simulink model "SAC_RW"  (R2020b)
settings: Solver=ode4  StartTime=0.0  StopTime=T  FixedStep=s  RelTol=1e-3  EnableMultiTasking=on
values from neighbouring files (symbols this model uses):
  A = [zeros(3,3), eye(3); (-1*(wn)^2)*eye(3),-2*zeta*wn*eye(3)]    [ini_SAC.m]    (also in ini_SACRW.m = [zeros(3,3), eye(3); (-1*(wnn)^2)*eye(3),-2*zetaa*wnn*eye(3))
  a1_B = [1,0,0]'    [ini_SAC.m]    (also in ini_SACRW.m)
  a2_B = [0,1,0]'    [ini_SAC.m]    (also in ini_SACRW.m)
  a3_B = [0,0,1]'    [ini_SAC.m]    (also in ini_SACRW.m)
  alpha = 1    [ini_SAC.m]    (also in ini_SACRW.m)
  B = [zeros(3,3);(wn^2)*eye(3)]    [ini_SAC.m]    (also in ini_SACRW.m = [zeros(3,3);(wnn^2)*eye(3)])
  C = [eye(6)]    [ini_SAC.m]    (also in ini_SACRW.m)
  D = [zeros(6,3)]    [ini_SAC.m]    (also in ini_SACRW.m)
  gIE = 1e5*(eye(3))    [ini_SAC.m]    (also in ini_SACRW.m = 1e3*(eye(3)))
  gIU = 1e3*(eye(3))    [ini_SAC.m]    (also in ini_SACRW.m)
  gIX = 1e3*(eye(6))    [ini_SAC.m]    (also in ini_SACRW.m)
  gPE = 1e5*(eye(3))    [ini_SAC.m]    (also in ini_SACRW.m = 1e3*(eye(3)))
  gPU = 1e3*(eye(3))    [ini_SAC.m]    (also in ini_SACRW.m)
  gPX = 1e3*(eye(6))    [ini_SAC.m]    (also in ini_SACRW.m)
  Jsc = [114 0 0;0 86 0;0 0 87]    [ini_SAC.m]    (also in ini_SACRW.m = 1*[114 0 0;0 86 0;0 0 87])
  Jsc_inv = Jsc^-1    [ini_SAC.m]    (also in ini_SACRW.m)
  q_d = [0 0 0 1]'    [ini_SAC.m]    (also in ini_SACRW.m)
  qsc_I_ini = [a(1)*sin(phiR/2) a(2)*sin(phiR/2) a(3)*sin(phiR/2) cos(phiR/2)]    [ini_SACRW.m]
  r_I_ini = [-0.1 0.5 1.0]    [ini_SAC.m]
  r_I_ini_dot = [0 0 0]    [ini_SACRW.m]
  r_I_ini_pos = (qsc_I_ini(1:3)/qsc_I_ini(4))    [ini_SACRW.m]
  rw_t = 0.01    [ini_SAC.m]    (also in ini_SACRW.m)
undefined symbols (not defined in the file or in its folder): gammaE, gammaU, gammaX, K
libraries: simulink_extras x3
settings Model: Creator=hoomanrajaee  LastModifiedBy=Graham Stokes
settings DataIOCC: LimitDataPoints=on  SaveFormat=Array  SignalLoggingSaveFormat=ModelDataLogs  ReturnWorkspaceOutputs=off
settings OptimizationCC: LifeSpan=inf
settings DebuggingCC: UnderspecifiedInitializationDetection=Classic  MergeDetectMultiDrivingBlocksExec=none  SolverPrmCheckMsg=warning  MultiTaskDSMMsg=warning  MultiTaskCondExecSysMsg=none  AllowSymbolicDim=off  StateNameClashWarn=warning  SFUnexpectedBacktrackingDiag=warning  SFNoUnconditionalDefaultTransitionDiag=warning  UnderSpecifiedDimensionMsg=warning  ArithmeticOperatorsInVariantConditions=warning
settings HardwareCC: ProdBitPerPointer=32  ProdBitPerSizeT=32  ProdBitPerPtrDiffT=32  ProdLargestAtomicFloat=None  ProdIntDivRoundTo=Undefined  ProdEndianess=Unspecified  ProdWordSize=32  ProdHWDeviceType=32-bit Generic
settings ModelReferenceCC: PropagateSignalLabelsOutOfModel=off
settings SFSimCC: SimUseLocalCustomCode=off  CustomCodeUndefinedFunction=UseInterfaceOnly
settings RTWCC: RTWUseLocalCustomCode=off
settings CodeAppCC: StateflowObjectComments=on
settings GRTTargetCC: TargetLangStandard=C89/C90 (ANSI)
settings ConfigComp: CovMetricSettings=dw  CovSaveCumulativeToWorkspaceVar=on  CovSaveSingleToWorkspaceVar=on  CovExternalEMLEnable=off

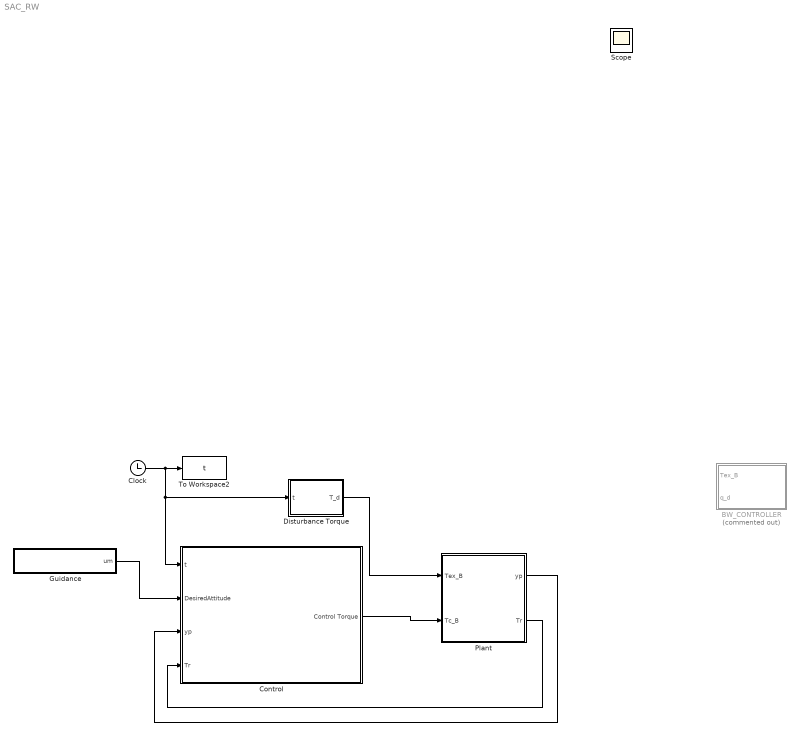
== system SAC_RW ==
  BW_CONTROLLER : Subsystem  Commented=on
  Clock : Clock
  Control : Subsystem
  Disturbance Torque : MATLAB Function  TreatAsAtomicUnit=on
  "Guidance " : Subsystem
  Plant : Subsystem
  To Workspace2 : ToWorkspace  VariableName=t  SampleTime=-1
  Scope : Scope
  wires:
  Clock/1 -> Disturbance Torque/1(t), Control/1(t), To Workspace2/1
  "Guidance "/1(um) -> Control/2(DesiredAttitude)
  Control/1(Control Torque) -> Plant/2(Tc_B)
  Plant/1("yp ") -> Control/3(yp)
  Plant/2("Tr ") -> Control/4(Tr)
  Disturbance Torque/1(T_d) -> Plant/1(Tex_B)

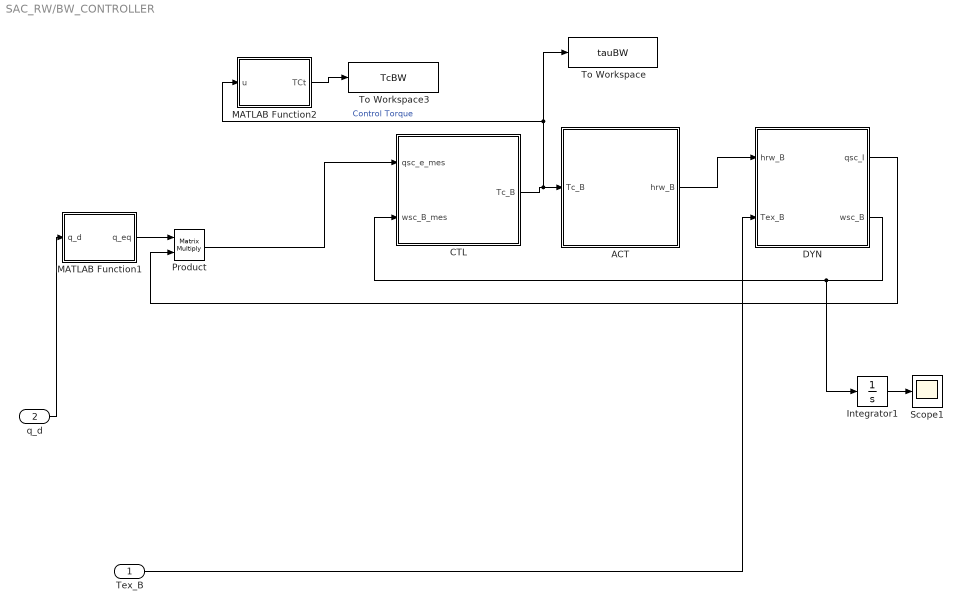
== system SAC_RW/BW_CONTROLLER ==
  Tex_B : Inport
  q_d : Inport  Port=2
  ACT : Subsystem
  CTL : Subsystem
  DYN : Subsystem
  Integrator1 : Integrator  InitialCondition=r_I_ini
  MATLAB Function1 : MATLAB Function  TreatAsAtomicUnit=on
  MATLAB Function2 : MATLAB Function  TreatAsAtomicUnit=on
  Product : Product  Multiplication=Matrix(*)
  Scope1 : Scope
  To Workspace : ToWorkspace  VariableName=tauBW  SaveFormat=Timeseries  SampleTime=-1
  To Workspace3 : ToWorkspace  VariableName=TcBW  SaveFormat=Timeseries  SampleTime=-1
  wires:
  ACT/1(hrw_B) -> DYN/1(hrw_B)
  MATLAB Function1/1(q_eq) -> Product/1
  DYN/1(qsc_I) -> Product/2
  Product/1 -> CTL/1(qsc_e_mes)
  q_d/1 -> MATLAB Function1/1(q_d)
  Tex_B/1 -> DYN/2(Tex_B)
  CTL/1(Tc_B) -> To Workspace/1, MATLAB Function2/1(u), ACT/1(Tc_B)  "Control Torque"
  MATLAB Function2/1(TCt) -> To Workspace3/1
  Integrator1/1 -> Scope1/1
  DYN/2(wsc_B) -> Integrator1/1, CTL/2(wsc_B_mes)

== system SAC_RW/Control ==
  t : Inport
  DesiredAttitude : Inport  Port=2
  yp : Inport  Port=3
  Tr : Inport  Port=4
  ADAPTIVE CONTROLLER : Subsystem
      settings: AttributesFormatString=Adaptive Controller
  MODEL PLANT : Subsystem
  Sum : Sum  Inputs=|+-
  To Workspace : ToWorkspace  VariableName=tau  SaveFormat=Timeseries  SampleTime=-1
  Control Torque : Outport
  wires:
  DesiredAttitude/1 -> ADAPTIVE CONTROLLER/4(um1), MODEL PLANT/1(DesiredAttitude)
  MODEL PLANT/2(ym) -> Sum/1
  Tr/1 -> ADAPTIVE CONTROLLER/2(Tr)
  ADAPTIVE CONTROLLER/1(tau) -> To Workspace/1, Control Torque/1  "Control Torque"
  yp/1 -> Sum/2
  Sum/1 -> ADAPTIVE CONTROLLER/1(ey1)  "ey"
  MODEL PLANT/1(xm) -> ADAPTIVE CONTROLLER/3(xm1)
  t/1 -> MODEL PLANT/2(In2)

== system SAC_RW/Guidance  ==
  MRP : MATLAB Function  TreatAsAtomicUnit=on
  To Workspace : ToWorkspace  VariableName=um  SaveFormat=Timeseries  SampleTime=-1
  q_d1 : Constant  Value=q_d
  um : Outport
  wires:
  MRP/1(r) -> To Workspace/1, um/1  "um"
  q_d1/1 -> MRP/1(qsc_I_sign)

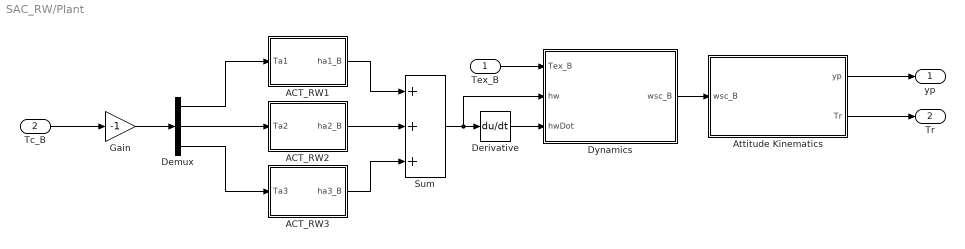
== system SAC_RW/Plant ==
  Tex_B : Inport
  Tc_B : Inport  Port=2
  ACT_RW1 : Subsystem
  ACT_RW2 : Subsystem
  ACT_RW3 : Subsystem
  Attitude Kinematics : Subsystem
  Demux : Demux  Outputs=3
  Derivative : Derivative
  Dynamics : Subsystem
  Gain : Gain  Gain=-1
  Sum : Sum  Inputs=+++
  "yp " : Outport
  "Tr " : Outport  Port=2
  wires:
  Attitude Kinematics/2(Tr) -> "Tr "/1
  Attitude Kinematics/1(yp) -> "yp "/1
  Demux/3 -> ACT_RW3/1(Ta3)
  ACT_RW2/1(ha2_B) -> Sum/2
  Demux/1 -> ACT_RW1/1(Ta1)
  ACT_RW1/1(ha1_B) -> Sum/1
  ACT_RW3/1(ha3_B) -> Sum/3
  Sum/1 -> Derivative/1, Dynamics/2(hw)
  Demux/2 -> ACT_RW2/1(Ta2)
  Derivative/1 -> Dynamics/3(hwDot)
  Tex_B/1 -> Dynamics/1(Tex_B)
  Tc_B/1 -> Gain/1
  Dynamics/1(wsc_B) -> Attitude Kinematics/1(wsc_B)
  Gain/1 -> Demux/1

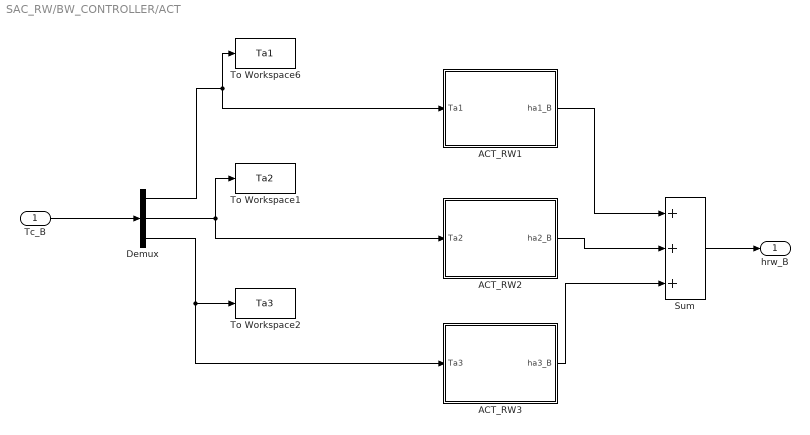
== system SAC_RW/BW_CONTROLLER/ACT ==
  Tc_B : Inport
  ACT_RW1 : Subsystem
  ACT_RW2 : Subsystem
  ACT_RW3 : Subsystem
  Demux : Demux  Outputs=3
  Sum : Sum  Inputs=+++
  To Workspace1 : ToWorkspace  VariableName=Ta2  SampleTime=-1
  To Workspace2 : ToWorkspace  VariableName=Ta3  SampleTime=-1
  To Workspace6 : ToWorkspace  VariableName=Ta1  SampleTime=-1
  hrw_B : Outport
  wires:
  ACT_RW1/1(ha1_B) -> Sum/1
  Sum/1 -> hrw_B/1
  Demux/1 -> ACT_RW1/1(Ta1), To Workspace6/1
  Demux/2 -> To Workspace1/1, ACT_RW2/1(Ta2)
  Demux/3 -> To Workspace2/1, ACT_RW3/1(Ta3)
  ACT_RW2/1(ha2_B) -> Sum/2
  ACT_RW3/1(ha3_B) -> Sum/3
  Tc_B/1 -> Demux/1

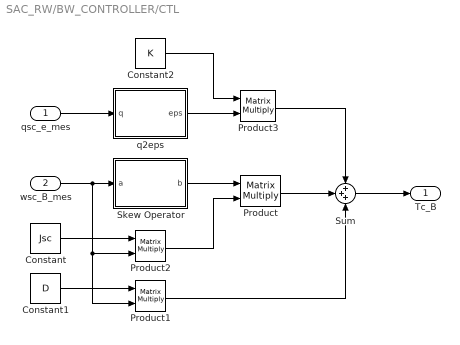
== system SAC_RW/BW_CONTROLLER/CTL ==
  qsc_e_mes : Inport
  wsc_B_mes : Inport  Port=2
  Constant : Constant  Value=Jsc
  Constant1 : Constant  Value=D
  Constant2 : Constant  Value=K
  Product{,1..3} (4 alike) : Product  Multiplication=Matrix(*)
  Skew Operator : MATLAB Function  TreatAsAtomicUnit=on
  Sum : Sum  Inputs=+++
  q2eps : MATLAB Function  TreatAsAtomicUnit=on
  Tc_B : Outport
  wires:
  wsc_B_mes/1 -> Skew Operator/1(a), Product2/2, Product1/2
  Skew Operator/1(b) -> Product/1
  Product2/1 -> Product/2
  Product3/1 -> Sum/1
  qsc_e_mes/1 -> q2eps/1(q)
  q2eps/1(eps) -> Product3/2
  Sum/1 -> Tc_B/1
  Product1/1 -> Sum/3
  Constant/1 -> Product2/1
  Constant1/1 -> Product1/1
  Constant2/1 -> Product3/1
  Product/1 -> Sum/2

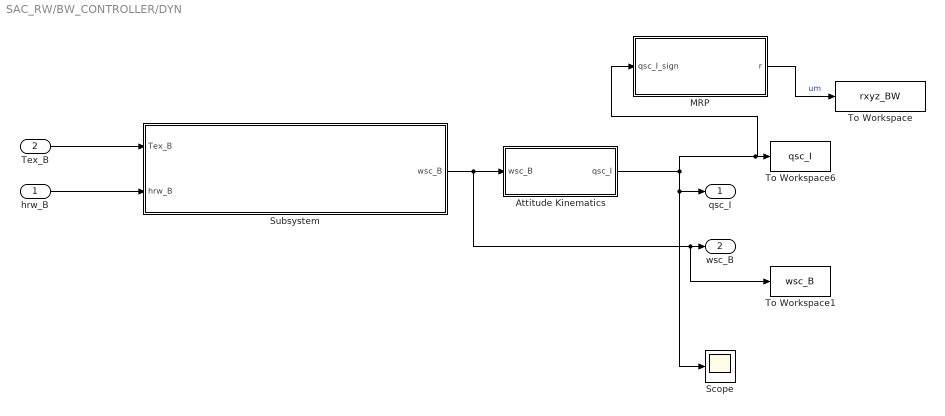
== system SAC_RW/BW_CONTROLLER/DYN ==
  hrw_B : Inport
  Tex_B : Inport  Port=2
  Attitude Kinematics : Subsystem
  MRP : MATLAB Function  TreatAsAtomicUnit=on
  Scope : Scope
  Subsystem : Subsystem
  To Workspace : ToWorkspace  VariableName=rxyz_BW  SaveFormat=Timeseries  SampleTime=-1
  To Workspace1 : ToWorkspace  VariableName=wsc_B  SampleTime=-1
  To Workspace6 : ToWorkspace  VariableName=qsc_I  SampleTime=-1
  qsc_I : Outport
  wsc_B : Outport  Port=2
  wires:
  Attitude Kinematics/1(qsc_I) -> Scope/1, qsc_I/1, MRP/1(qsc_I_sign), To Workspace6/1
  Subsystem/1(wsc_B) -> To Workspace1/1, wsc_B/1, Attitude Kinematics/1(wsc_B)
  Tex_B/1 -> Subsystem/1(Tex_B)
  hrw_B/1 -> Subsystem/2(hrw_B)
  MRP/1(r) -> To Workspace/1  "um"

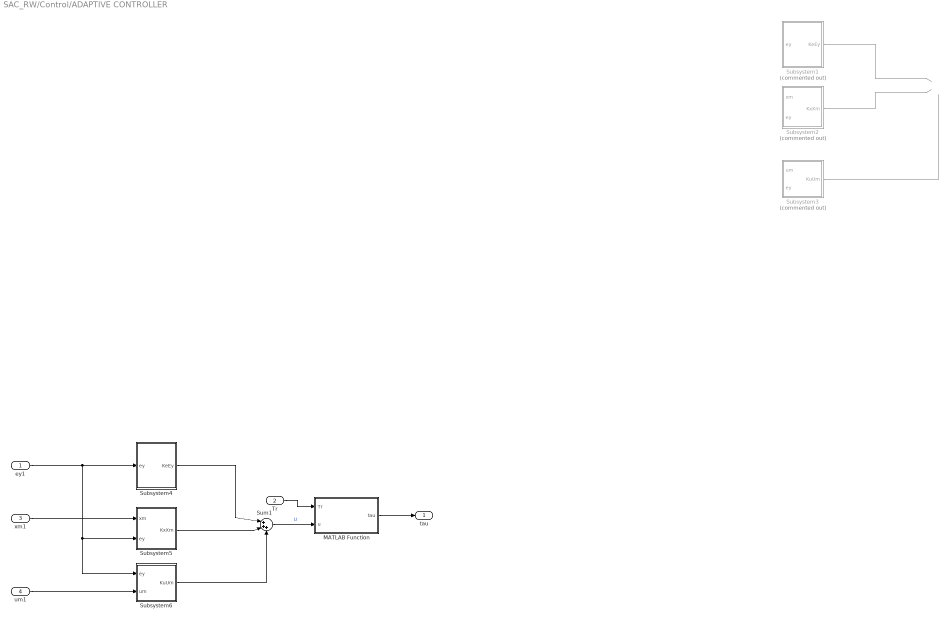
== system SAC_RW/Control/ADAPTIVE CONTROLLER ==
  ey1 : Inport
  Tr : Inport  Port=2
  xm1 : Inport  Port=3
  um1 : Inport  Port=4
  MATLAB Function : MATLAB Function  TreatAsAtomicUnit=on
  Subsystem1 : Subsystem  Commented=on
  Subsystem2 : Subsystem  Commented=on
  Subsystem3 : Subsystem  Commented=on
  Subsystem4 : Subsystem
  Subsystem5 : Subsystem
  Subsystem6 : Subsystem
  Sum1 : Sum  Inputs=|+++
  tau : Outport
  wires:
  Tr/1 -> MATLAB Function/1(Tr)
  Sum1/1 -> MATLAB Function/2(u)  "U"
  MATLAB Function/1(tau) -> tau/1
  Subsystem5/1(KxXm) -> Sum1/2
  Subsystem4/1(KeEy) -> Sum1/1
  Subsystem6/1(KuUm) -> Sum1/3
  um1/1 -> Subsystem6/2(um)
  xm1/1 -> Subsystem5/1(xm)
  ey1/1 -> Subsystem4/1(ey), Subsystem6/1(ey), Subsystem5/2(ey)
  Subsystem2/1(KxXm) -> ?
  Subsystem3/1(KuUm) -> ?
  Subsystem1/1(KeEy) -> ?

== system SAC_RW/Control/MODEL PLANT ==
  DesiredAttitude : Inport
  In2 : Inport  Port=2
  Constant : Constant  Value=alpha
  MATLAB Function : MATLAB Function  TreatAsAtomicUnit=on
  Scope : Scope
  State Space Model : Subsystem
  State-Space : StateSpace  Commented=on  A=A  B=B  C=C  D=D  InitialCondition=[r_I_ini(1);r_I_ini(2);r_I_ini(3);0;0;0]
  xm : Outport
  ym : Outport  Port=2
  wires:
  MATLAB Function/1(ym) -> ym/1
  Constant/1 -> MATLAB Function/2(alpha)
  State Space Model/1(Xm) -> xm/1, Scope/1, MATLAB Function/1(Xm)
  DesiredAttitude/1 -> State Space Model/1(DesiredAttitude)  "U"
  In2/1 -> State Space Model/2(In2)

== system SAC_RW/Plant/ACT_RW1 ==
  Ta1 : Inport
  Constant1 : Constant  Value=a1_B
  Integrator : Integrator
  Product1 : Product
  Transfer Fcn (with initial states) : simulink_extras/Additional Linear/Transfer Fcn (with initial states)  N=[1]  D=[rw_t 1]  X0=.5
  ha1_B : Outport
  wires:
  Product1/1 -> ha1_B/1
  Integrator/1 -> Product1/1
  Constant1/1 -> Product1/2
  Ta1/1 -> Transfer Fcn (with initial states)/1
  Transfer Fcn (with initial states)/1 -> Integrator/1

== system SAC_RW/Plant/ACT_RW2 ==
  Ta2 : Inport
  Constant1 : Constant  Value=a2_B
  Integrator : Integrator
  Product1 : Product
  Transfer Fcn (with initial states) : simulink_extras/Additional Linear/Transfer Fcn (with initial states)  N=[1]  D="[rw_t  1]"  X0=.5
  ha2_B : Outport
  wires:
  Constant1/1 -> Product1/2
  Product1/1 -> ha2_B/1
  Integrator/1 -> Product1/1
  Ta2/1 -> Transfer Fcn (with initial states)/1  "Tcmd"
  Transfer Fcn (with initial states)/1 -> Integrator/1

== system SAC_RW/Plant/ACT_RW3 ==
  Ta3 : Inport
  Constant1 : Constant  Value=a3_B
  Integrator : Integrator
  Product1 : Product
  Transfer Fcn (with initial states) : simulink_extras/Additional Linear/Transfer Fcn (with initial states)  N=[1]  D="[rw_t  1]"  X0=.5
  ha3_B : Outport
  wires:
  Constant1/1 -> Product1/2
  Product1/1 -> ha3_B/1
  Integrator/1 -> Product1/1
  Ta3/1 -> Transfer Fcn (with initial states)/1  "Tcmd"
  Transfer Fcn (with initial states)/1 -> Integrator/1

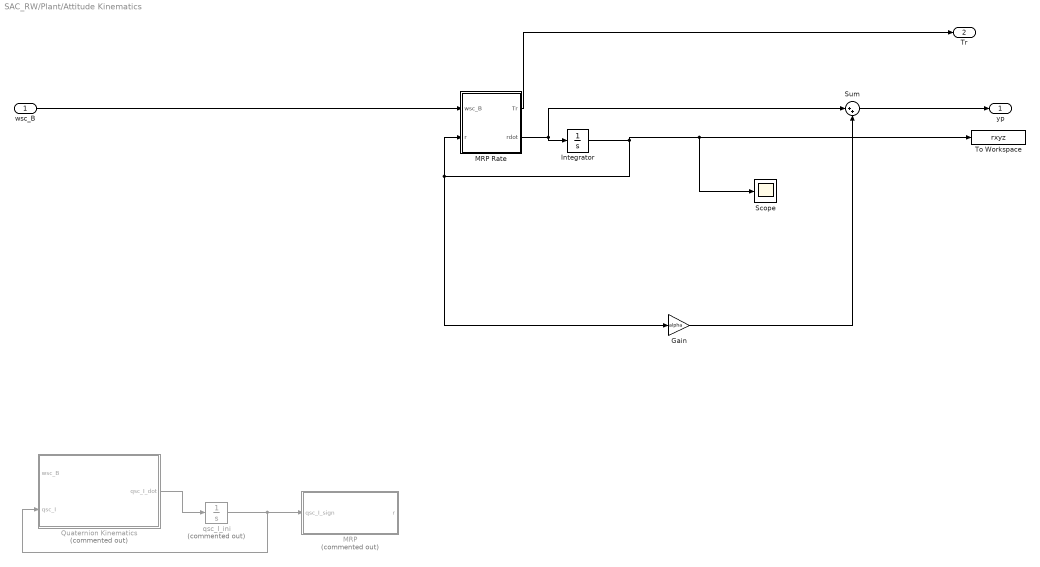
== system SAC_RW/Plant/Attitude Kinematics ==
  wsc_B : Inport
  Gain : Gain  Gain=alpha
  Integrator : Integrator  InitialCondition=r_I_ini_pos
  MRP : MATLAB Function  Commented=on  TreatAsAtomicUnit=on
  MRP Rate : MATLAB Function  TreatAsAtomicUnit=on
  Quaternion Kinematics : MATLAB Function  Commented=on  TreatAsAtomicUnit=on
  Scope : Scope
  Sum : Sum  Inputs=|++
  To Workspace : ToWorkspace  VariableName=rxyz  SaveFormat=Timeseries  SampleTime=-1
  qsc_I_ini : Integrator  Commented=on  InitialCondition=qsc_I_ini
  yp : Outport
  Tr : Outport  Port=2
  wires:
  MRP Rate/2(rdot) -> Sum/1, Integrator/1
  Sum/1 -> yp/1
  Gain/1 -> Sum/2
  MRP Rate/1(Tr) -> Tr/1
  wsc_B/1 -> MRP Rate/1(wsc_B)
  Quaternion Kinematics/1(qsc_I_dot) -> qsc_I_ini/1
  qsc_I_ini/1 -> MRP/1(qsc_I_sign), Quaternion Kinematics/2(qsc_I)
  Integrator/1 -> Gain/1, MRP Rate/2(r), Scope/1, To Workspace/1

== system SAC_RW/Plant/Dynamics ==
  Tex_B : Inport
  hw : Inport  Port=2
  hwDot : Inport  Port=3
  Constant1 : Constant  Value=Jsc
  Integrator : Integrator  InitialCondition=[0 0 0]';
  MATLAB Function : MATLAB Function  TreatAsAtomicUnit=on
  To Workspace : ToWorkspace  VariableName=w_sc  SaveFormat=Timeseries  SampleTime=-1
  wsc_B : Outport
  wires:
  Integrator/1 -> MATLAB Function/2(wsc_B), To Workspace/1, wsc_B/1
  Constant1/1 -> MATLAB Function/3(Jsc)
  MATLAB Function/1(angularAcceleration) -> Integrator/1
  Tex_B/1 -> MATLAB Function/1(Tex_B)
  hw/1 -> MATLAB Function/4(hw)
  hwDot/1 -> MATLAB Function/5(hwDot)

== system SAC_RW/BW_CONTROLLER/ACT/ACT_RW1 ==
  Ta1 : Inport
  Constant1 : Constant  Value=a1_B
  Integrator : Integrator
  Product1 : Product
  ha1_B : Outport
  wires:
  Ta1/1 -> Integrator/1
  Product1/1 -> ha1_B/1
  Integrator/1 -> Product1/1
  Constant1/1 -> Product1/2

== system SAC_RW/BW_CONTROLLER/ACT/ACT_RW2 ==
  Ta2 : Inport
  Constant1 : Constant  Value=a2_B
  Integrator : Integrator
  Product1 : Product
  ha2_B : Outport
  wires:
  Constant1/1 -> Product1/2
  Product1/1 -> ha2_B/1
  Integrator/1 -> Product1/1
  Ta2/1 -> Integrator/1

== system SAC_RW/BW_CONTROLLER/ACT/ACT_RW3 ==
  Ta3 : Inport
  Constant1 : Constant  Value=a3_B
  Integrator : Integrator
  Product1 : Product
  ha3_B : Outport
  wires:
  Constant1/1 -> Product1/2
  Product1/1 -> ha3_B/1
  Integrator/1 -> Product1/1
  Ta3/1 -> Integrator/1

== system SAC_RW/BW_CONTROLLER/DYN/Attitude Kinematics ==
  wsc_B : Inport
  Quaternion Kinematics : MATLAB Function  TreatAsAtomicUnit=on
  Quaternion Normalization : MATLAB Function  TreatAsAtomicUnit=on
  Quaternion Sign Check : MATLAB Function  TreatAsAtomicUnit=on
  qsc_I_ini : Integrator  InitialCondition=qsc_I_ini
  qsc_I : Outport
  wires:
  Quaternion Kinematics/1(qsc_I_dot) -> qsc_I_ini/1
  wsc_B/1 -> Quaternion Kinematics/1(wsc_B)
  Quaternion Sign Check/1(qsc_I_sign) -> Quaternion Kinematics/2(qsc_I), qsc_I/1
  Quaternion Normalization/1(qsc_I_norm) -> Quaternion Sign Check/1(qsc_I)
  qsc_I_ini/1 -> Quaternion Normalization/1(qsc_I)

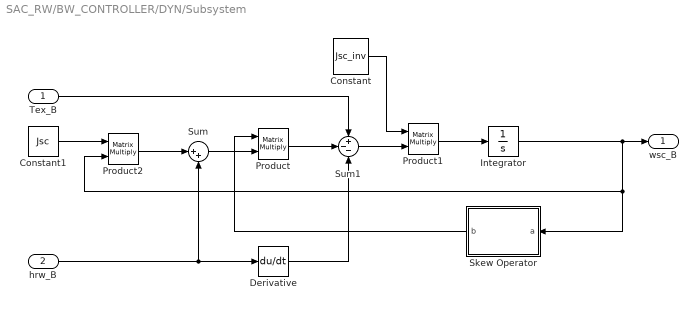
== system SAC_RW/BW_CONTROLLER/DYN/Subsystem ==
  Tex_B : Inport
  hrw_B : Inport  Port=2
  Constant : Constant  Value=Jsc_inv
  Constant1 : Constant  Value=Jsc
  Derivative : Derivative
  Integrator : Integrator
  Product : Product  Multiplication=Matrix(*)
  Product1 : Product  Multiplication=Matrix(*)
  Product2 : Product  Multiplication=Matrix(*)
  Skew Operator : MATLAB Function  TreatAsAtomicUnit=on
  Sum : Sum  Inputs=|++
  Sum1 : Sum  Inputs=+--
  wsc_B : Outport
  wires:
  hrw_B/1 -> Derivative/1, Sum/2
  Integrator/1 -> wsc_B/1, Skew Operator/1(a), Product2/2
  Product2/1 -> Sum/1
  Product/1 -> Sum1/2
  Derivative/1 -> Sum1/3
  Tex_B/1 -> Sum1/1
  Product1/1 -> Integrator/1
  Sum1/1 -> Product1/2
  Constant/1 -> Product1/1
  Skew Operator/1(b) -> Product/1
  Sum/1 -> Product/2
  Constant1/1 -> Product2/1

== system SAC_RW/Control/ADAPTIVE CONTROLLER/Subsystem1 ==
  ey : Inport
  Add : Sum
  Constant1 : Constant  Value=gammaE
  Integrator : Integrator
  KIE : MATLAB Function  TreatAsAtomicUnit=on
  KPE : MATLAB Function  TreatAsAtomicUnit=on
  MATLAB Function : MATLAB Function  Commented=on  TreatAsAtomicUnit=on
  Product : Product  Multiplication=Matrix(*)
  KeEy : Outport
  wires:
  ey/1 -> Product/2, KPE/1(ey), KIE/1(ey)
  KPE/1(Kpe) -> Add/1
  KIE/1(KIe) -> Integrator/1
  Constant1/1 -> KPE/2(gammaE), KIE/2(gammaE)
  Product/1 -> KeEy/1  "KeEy"
  Integrator/1 -> Add/2
  Add/1 -> Product/1

== system SAC_RW/Control/ADAPTIVE CONTROLLER/Subsystem2 ==
  xm : Inport
  ey : Inport  Port=2
  Add : Sum
  Constant1 : Constant  Value=gammaX
  Integrator : Integrator
  KIX : MATLAB Function  TreatAsAtomicUnit=on
  KPE : MATLAB Function  TreatAsAtomicUnit=on
  MATLAB Function : MATLAB Function  Commented=on  TreatAsAtomicUnit=on
  Product : Product  Multiplication=Matrix(*)
  KxXm : Outport
  wires:
  ey/1 -> KPE/1(ey), KIX/1(ey)
  xm/1 -> Product/2, KIX/2(xm), KPE/2(xm)
  Add/1 -> Product/1
  Integrator/1 -> Add/2
  KPE/1(Kpx) -> Add/1
  Constant1/1 -> KPE/3(gammaX), KIX/3(gammaX)
  Product/1 -> KxXm/1  "KXxm"
  KIX/1(KIx) -> Integrator/1

== system SAC_RW/Control/ADAPTIVE CONTROLLER/Subsystem3 ==
  um : Inport
  ey : Inport  Port=2
  Add : Sum
  Constant1 : Constant  Value=gammaU
  Integrator : Integrator
  KIu : MATLAB Function  TreatAsAtomicUnit=on
  KPE : MATLAB Function  TreatAsAtomicUnit=on
  MATLAB Function : MATLAB Function  Commented=on  TreatAsAtomicUnit=on
  Product : Product  Multiplication=Matrix(*)
  KuUm : Outport
  wires:
  Product/1 -> KuUm/1  "KuUm"
  KIu/1(KIu) -> Integrator/1
  ey/1 -> KPE/1(ey), KIu/1(ey)
  KPE/1(KPu) -> Add/1
  Integrator/1 -> Add/2
  Constant1/1 -> KIu/3(gammaU), KPE/3(gammaU)
  um/1 -> Product/2, KPE/2(um), KIu/2(um)
  Add/1 -> Product/1

== system SAC_RW/Control/ADAPTIVE CONTROLLER/Subsystem4 ==
  ey : Inport
  Add : Sum
  Constant1 : Constant  Value=gPE
  Constant2 : Constant  Value=gIE
  Integrator : Integrator
  KIE : MATLAB Function  TreatAsAtomicUnit=on
  KPE : MATLAB Function  TreatAsAtomicUnit=on
  Product : Product  Multiplication=Matrix(*)
  KeEy : Outport
  wires:
  ey/1 -> KPE/1(ey), KIE/1(ey), Product/2
  KPE/1(Kpe) -> Add/1
  KIE/1(KIe) -> Integrator/1
  Constant1/1 -> KPE/2(gPE)
  Product/1 -> KeEy/1  "KeEy"
  Integrator/1 -> Add/2
  Add/1 -> Product/1
  Constant2/1 -> KIE/2(gIE)

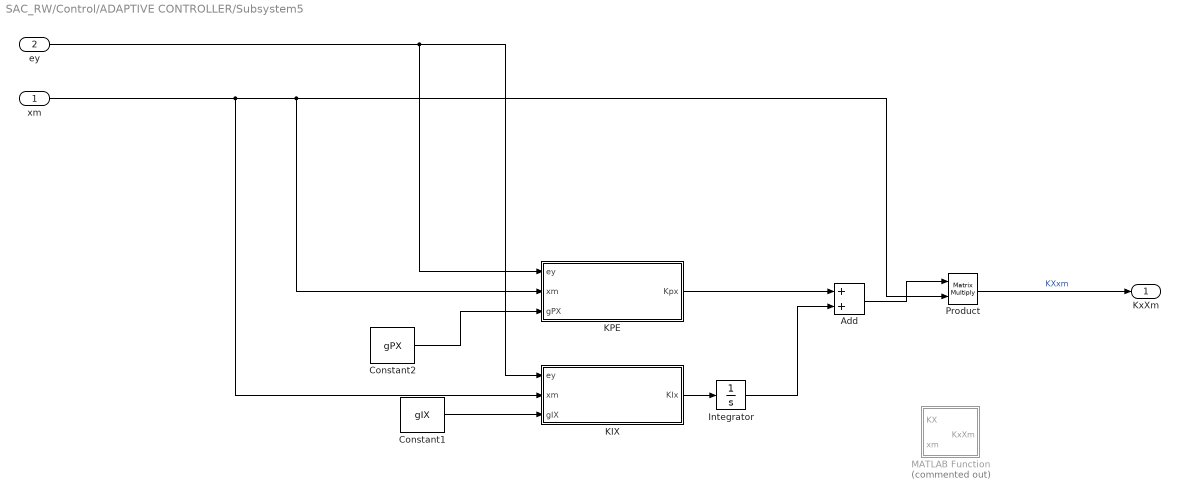
== system SAC_RW/Control/ADAPTIVE CONTROLLER/Subsystem5 ==
  xm : Inport
  ey : Inport  Port=2
  Add : Sum
  Constant1 : Constant  Value=gIX
  Constant2 : Constant  Value=gPX
  Integrator : Integrator
  KIX : MATLAB Function  TreatAsAtomicUnit=on
  KPE : MATLAB Function  TreatAsAtomicUnit=on
  MATLAB Function : MATLAB Function  Commented=on  TreatAsAtomicUnit=on
  Product : Product  Multiplication=Matrix(*)
  KxXm : Outport
  wires:
  ey/1 -> KPE/1(ey), KIX/1(ey)
  xm/1 -> KPE/2(xm), Product/2, KIX/2(xm)
  Add/1 -> Product/1
  Integrator/1 -> Add/2
  KPE/1(Kpx) -> Add/1
  Constant1/1 -> KIX/3(gIX)
  Product/1 -> KxXm/1  "KXxm"
  KIX/1(KIx) -> Integrator/1
  Constant2/1 -> KPE/3(gPX)

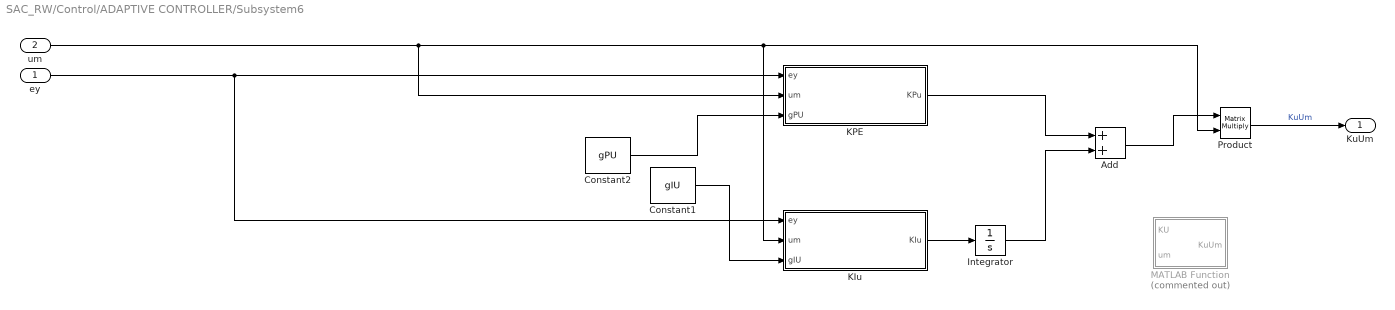
== system SAC_RW/Control/ADAPTIVE CONTROLLER/Subsystem6 ==
  ey : Inport
  um : Inport  Port=2
  Add : Sum
  Constant1 : Constant  Value=gIU
  Constant2 : Constant  Value=gPU
  Integrator : Integrator
  KIu : MATLAB Function  TreatAsAtomicUnit=on
  KPE : MATLAB Function  TreatAsAtomicUnit=on
  MATLAB Function : MATLAB Function  Commented=on  TreatAsAtomicUnit=on
  Product : Product  Multiplication=Matrix(*)
  KuUm : Outport
  wires:
  Product/1 -> KuUm/1  "KuUm"
  KIu/1(KIu) -> Integrator/1
  ey/1 -> KPE/1(ey), KIu/1(ey)
  KPE/1(KPu) -> Add/1
  Integrator/1 -> Add/2
  Constant1/1 -> KIu/3(gIU)
  um/1 -> KIu/2(um), Product/2, KPE/2(um)
  Add/1 -> Product/1
  Constant2/1 -> KPE/3(gPU)

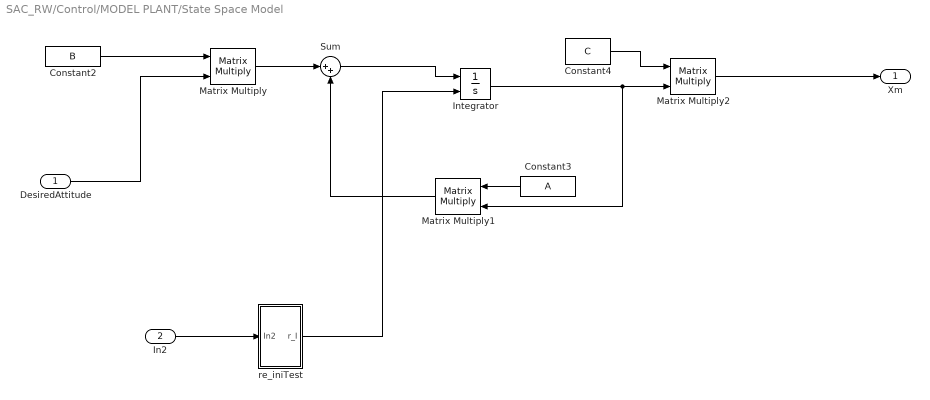
== system SAC_RW/Control/MODEL PLANT/State Space Model ==
  DesiredAttitude : Inport
  In2 : Inport  Port=2
  Constant2 : Constant  Value=B
  Constant3 : Constant  Value=A
  Constant4 : Constant  Value=C
  Integrator : Integrator  InitialConditionSource=external
  Matrix Multiply : Product  Multiplication=Matrix(*)
  Matrix Multiply1 : Product  Multiplication=Matrix(*)
  Matrix Multiply2 : Product  Multiplication=Matrix(*)
  Sum : Sum  Inputs=|++
  re_iniTest : Subsystem
  Xm : Outport
  wires:
  Matrix Multiply/1 -> Sum/1
  Integrator/1 -> Matrix Multiply2/2, Matrix Multiply1/2
  Sum/1 -> Integrator/1
  DesiredAttitude/1 -> Matrix Multiply/2
  Constant4/1 -> Matrix Multiply2/1
  Constant2/1 -> Matrix Multiply/1
  Matrix Multiply1/1 -> Sum/2
  Constant3/1 -> Matrix Multiply1/1
  Matrix Multiply2/1 -> Xm/1
  In2/1 -> re_iniTest/1(In2)
  re_iniTest/1(r_I) -> Integrator/2

== system SAC_RW/Control/MODEL PLANT/State Space Model/re_iniTest ==
  In2 : Inport
  Constant1 : Constant  Value=r_I_ini_pos
  Constant5 : Constant  Value=r_I_ini_dot
  MATLAB Function : MATLAB Function  TreatAsAtomicUnit=on
  r_I : Outport
  wires:
  In2/1 -> MATLAB Function/1(t)
  Constant1/1 -> MATLAB Function/2(r_I_ini_pos)
  MATLAB Function/1(r_I) -> r_I/1
  Constant5/1 -> MATLAB Function/3(r_I_ini_dot)

== matlab function SAC_RW/Control/MODEL PLANT/MATLAB Function ==
  data: Xm input; ym output; alpha input
function ym = parseY(Xm, alpha)
    
    %creates a 3X1 matrix of state output
    %Includes position and damping value--> similar to plant output
    ym = alpha*eye(3)*Xm(1:3) + Xm(4:6);
    
end

== matlab function SAC_RW/Control/ADAPTIVE CONTROLLER/Subsystem3/MATLAB Function ==
  data: KU input; um input; KuUm output
function  KuUm = fcn(KU, um)

KuUm = KU*um

end

== matlab function SAC_RW/Control/ADAPTIVE CONTROLLER/Subsystem2/MATLAB Function ==
  data: KX input; xm input; KxXm output
function  KxXm = KX(KX, xm)

KxXm = KX*xm

end

== matlab function SAC_RW/Plant/Attitude Kinematics/MRP ==
  data: qsc_I_sign input; r output
function r  = QuatToMRP(qsc_I_sign)
    q = qsc_I_sign; 
    r = zeros(3,1); 
    eps = zeros(3,1); 
    
    eps(1) = q(1);
    eps(2) = q(2); 
    eps(3) = q(3); 
    
    r = eps/(1+q(4)); 
end

== matlab function SAC_RW/Plant/Attitude Kinematics/MRP Rate ==
  data: Tr output; wsc_B input; r input; rdot output
function [Tr,rdot]= fcn(wsc_B,r)
        
    Tr = zeros(3,3); 
    Tr = 0.25*((1-transpose(r)*r)*eye(3)+2*skew(r)+2*r*transpose(r));
   
    TrInv = zeros(3,3); 
    TrInv = 4*(((1+transpose(r)*r)^-2)*(1-transpose(r)*r)*eye(3)-2*skew(r)+2*r*transpose(r));
    
    %set size of T(r) matrix 
    rdot = Tr*wsc_B; 
    
end

== matlab function SAC_RW/Plant/Attitude Kinematics/Quaternion Kinematics ==
  data: wsc_B input; qsc_I_dot output; qsc_I input
function qsc_I_dot  = qdot(wsc_B,qsc_I)

% ---------------------------------------------------------------
% qdot
% ---------------------------------------------------------------
% Description:
% Calculate the quaternion differential kinematics
% ---------------------------------------------------------------
% Inputs:
% qsc_I => quaternion (4 x 1 matrix)
% wsc_B => angular rates (3 x 1 matrix)
% ---------------------------------------------------------------
% Outputs:
% qsc_I_dot => quaternion derivatives (4 x 1 matrix) 
% ---------------------------------------------------------------
% Parameters:
% None
% ---------------------------------------------------------------
% Copyright:
% Steve Ulrich, 2020
% ---------------------------------------------------------------

%prealocating
qsc_I_dot = [0 0 0 0]';

% Equation 1.76 in the text book
qsc_I_dot(1:3) = (1/2)*(qsc_I(4)*eye(3)+skew(qsc_I(1:3)))*wsc_B;
qsc_I_dot(4) = (-1/2)*(qsc_I(1:3)')*wsc_B;

end

== matlab function SAC_RW/Plant/Dynamics/MATLAB Function ==
  data: Tex_B input; angularAcceleration output; wsc_B input; Jsc input; hw input; hwDot input
function angularAcceleration = EulerDynamics(Tex_B,wsc_B,Jsc,hw,hwDot)
%% Euler's Equation of Motion



J_b = Jsc;
wsc_BB = wsc_B;
T = Tex_B;
wsc_skew = skew(wsc_B);

angularAcceleration = inv(J_b)*(T-(wsc_skew*(J_b*wsc_BB + hw))- hwDot);


end

== matlab function SAC_RW/Disturbance Torque ==
  data: t input; T_d output
function T_d = Dist(t)

    mu = 398600.4418;
    RE = 6378.137; 
    a = RE + 728;
    n = sqrt(mu/a^3); 
    a0 = 10^-6*[-4.14 10.2 -5.07]';
    a1 = 10^-6.*[6.92 -9.05 3.40]';
    b1 = 10^-6.*[-8.77 1.33 7.56]'; 

    T_d = a0 + a1*cos(n*t) + b1*sin(n*t); 

end

== matlab function SAC_RW/Guidance /MRP ==
  data: qsc_I_sign input; r output
function r  = QuatToMRP(qsc_I_sign)
    q = qsc_I_sign; 
    r = zeros(3,1); 
    eps = zeros(3,1); 
    
    eps(1) = q(1);
    eps(2) = q(2); 
    eps(3) = q(3); 
    
    r = eps/(1+q(4)); 
    
end

== matlab function SAC_RW/BW_CONTROLLER/CTL/Skew Operator ==
  data: a input; b output
function b = skew(a)
%Skew calculates the 3x3 skew symetric matrix of a 3x1 vector

 if size(a) ~= [3 1]
     error('invalid vector dimesions')
 else
    b = [0 -a(3) a(2); a(3) 0 -a(1); -a(2) a(1) 0];
 end 

end

== matlab function SAC_RW/BW_CONTROLLER/CTL/q2eps ==
  data: q input; eps output
function eps = q2eps(q)
%extracts epsilon (the first three elements) from a quaternion q

if size(q) ~= [4 1]
    error('invalid vector dimesions')
else
    eps = q(1:3);
end

== matlab function SAC_RW/BW_CONTROLLER/DYN/Attitude Kinematics/Quaternion Kinematics ==
  data: wsc_B input; qsc_I_dot output; qsc_I input
function qsc_I_dot  = qdot(wsc_B,qsc_I)

% ---------------------------------------------------------------
% qdot
% ---------------------------------------------------------------
% Description:
% Calculate the quaternion differential kinematics
% ---------------------------------------------------------------
% Inputs:
% qsc_I => quaternion (4 x 1 matrix)
% wsc_B => angular rates (3 x 1 matrix)
% ---------------------------------------------------------------
% Outputs:
% qsc_I_dot => quaternion derivatives (4 x 1 matrix) 
% ---------------------------------------------------------------
% Parameters:
% None
% ---------------------------------------------------------------
% Copyright:
% Steve Ulrich, 2020
% ---------------------------------------------------------------

%prealocating
qsc_I_dot = [0 0 0 0]';

% Equation 1.76 in the text book
qsc_I_dot(1:3) = (1/2)*(qsc_I(4)*eye(3)+skew(qsc_I(1:3)))*wsc_B;
qsc_I_dot(4) = (-1/2)*(qsc_I(1:3)')*wsc_B;

end

== matlab function SAC_RW/BW_CONTROLLER/DYN/Attitude Kinematics/Quaternion Normalization ==
  data: qsc_I_norm output; qsc_I input
function qsc_I_norm  =  QUANORM(qsc_I)

% ---------------------------------------------------------------
% QUANORM
% ---------------------------------------------------------------
% Description:
% Quaternion normalization  
% ---------------------------------------------------------------
% Inputs:
% qsc_I => quaternions (4 x 1 matrix)
% ---------------------------------------------------------------
% Outputs:
% qsc_I_norm => normalized quaternions (4 x 1 matrix) 
% ---------------------------------------------------------------
% Parameters:
% None
% ---------------------------------------------------------------
% Copyright:
% Steve Ulrich, 2020
% ---------------------------------------------------------------

qsc_I_norm = zeros(4,1);

temp = qsc_I(1)*qsc_I(1) + qsc_I(2)*qsc_I(2) + qsc_I(3)*qsc_I(3) + qsc_I(4)*qsc_I(4);

qsc_I_norm(1) = qsc_I(1)/sqrt(temp);
qsc_I_norm(2) = qsc_I(2)/sqrt(temp);
qsc_I_norm(3) = qsc_I(3)/sqrt(temp);
qsc_I_norm(4) = qsc_I(4)/sqrt(temp);

== matlab function SAC_RW/BW_CONTROLLER/DYN/Attitude Kinematics/Quaternion Sign Check ==
  data: qsc_I_sign output; qsc_I input
function qsc_I_sign  = QUASIGN(qsc_I)

% ---------------------------------------------------------------
% QUASIGN
% ---------------------------------------------------------------
% Description:
% Changes the sign of all quaternion whenever q(4) is negative.
% Keeping q(4) positive ensures that the rotation is the shortest
% one (e.g., 160 deg around axis instead of 200 deg around -axis).
% ---------------------------------------------------------------
% Inputs:
% qsc_I => quaternions (4 x 1 matrix)
% ---------------------------------------------------------------
% Outputs:
% qsc_I_sign => quaternions with proper signs (4 x 1 matrix) 
% ---------------------------------------------------------------
% Parameters:
% None
% ---------------------------------------------------------------
% Copyright:
% Steve Ulrich, 2020
% ---------------------------------------------------------------


qsc_I_sign = zeros(4,1);

 if qsc_I(4) < 0.0
    for k=1:4
       qsc_I_sign(k) = -qsc_I(k);
    end;
 else
    for k=1:4
       qsc_I_sign(k) = qsc_I(k);
    end;
 end;

== matlab function SAC_RW/BW_CONTROLLER/DYN/Subsystem/Skew Operator ==
  data: a input; b output
function b = skew(a)
%Skew calculates the 3x3 skew symetric matrix of a 3x1 vector

 if size(a) ~= [3 1]
     error('invalid vector dimesions')
 else
    b = [0 -a(3) a(2); a(3) 0 -a(1); -a(2) a(1) 0];
 end 

end

== matlab function SAC_RW/BW_CONTROLLER/MATLAB Function1 ==
  data: q_d input; q_eq output
function q_eq = q_eq(q_d)

if size(q_d) ~= [4 1]
    error('invalid vector dimesions')
else
    q1=q_d(1);
    q2=q_d(2);
    q3=q_d(3);
    q4=q_d(4);

    %eqn 7 in assignment
    q_eq = [q4 q3 -q2 -q1; -q3 q4 q1 -q2; q2 -q1 q4 -q3; q1 q2 q3 q4];
end

== matlab function SAC_RW/BW_CONTROLLER/DYN/MRP ==
  data: qsc_I_sign input; r output
function r  = QuatToMRP(qsc_I_sign)
    q = qsc_I_sign; 
    r = zeros(3,1); 
    eps = zeros(3,1); 
    
    eps(1) = q(1);
    eps(2) = q(2); 
    eps(3) = q(3); 
    
    r = eps/(1+q(4)); 
end

== matlab function SAC_RW/Control/ADAPTIVE CONTROLLER/Subsystem4/KIE ==
  data: ey input; KIe output; gIE input
function KIe = KIE(ey,gIE)
    KIe = ey*(ey')*gIE;
end

== matlab function SAC_RW/Control/MODEL PLANT/State Space Model/re_iniTest/MATLAB Function ==
  data: t input; r_I_ini_pos input; r_I output; r_I_ini_dot input
function r_I = fcn(t, r_I_ini_pos, r_I_ini_dot)
    %r_I = [0 0 0 0 0 0]';
%     if(t>200) 
%         r0 = [1 .2 0.1];
%         r_I(1) = r0(1); 
%         r_I(2) = r0(2); 
%         r_I(3) = r0(3); 
%     else 
        r0 = r_I_ini_pos; 
        r0Dot = r_I_ini_dot; 
        r_I = [r0;r0Dot];
    %end 
end

== matlab function SAC_RW/BW_CONTROLLER/MATLAB Function2 ==
  data: u input; TCt output
function TCt = fcn(u)

TCt = abs(u); 

end

== matlab function SAC_RW/Control/ADAPTIVE CONTROLLER/Subsystem4/KPE ==
  data: ey input; Kpe output; gPE input
function Kpe = KPE(ey,gPE)
    Kpe = ey*(ey')*gPE;
end

== matlab function SAC_RW/Control/ADAPTIVE CONTROLLER/Subsystem5/KIX ==
  data: ey input; KIx output; xm input; gIX input
function KIx = KIX(ey, xm,gIX)
    KIx = (ey)*(xm')*gIX;
end

== matlab function SAC_RW/Control/ADAPTIVE CONTROLLER/Subsystem5/KPE ==
  data: ey input; Kpx output; xm input; gPX input
function Kpx = KPX(ey, xm,gPX)
    Kpx = (ey)*(xm')*gPX;
end

== matlab function SAC_RW/Control/ADAPTIVE CONTROLLER/Subsystem5/MATLAB Function ==
  data: KX input; xm input; KxXm output
function  KxXm = KX(KX, xm)

KxXm = KX*xm

end

== matlab function SAC_RW/Control/ADAPTIVE CONTROLLER/Subsystem6/KIu ==
  data: ey input; um input; KIu output; gIU input
function KIu = KIU(ey,um,gIU)
    KIu = ey*(um')*gIU;
end

== matlab function SAC_RW/Control/ADAPTIVE CONTROLLER/Subsystem6/KPE ==
  data: ey input; KPu output; um input; gPU input
function KPu = KPU(ey,um,gPU)
    KPu = ey*(um')*gPU;
end

== matlab function SAC_RW/Control/ADAPTIVE CONTROLLER/Subsystem6/MATLAB Function ==
  data: KU input; um input; KuUm output
function  KuUm = fcn(KU, um)

KuUm = KU*um

end

== matlab function SAC_RW/Control/ADAPTIVE CONTROLLER/Subsystem1/KIE ==
  data: ey input; KIe output; gammaE input
function KIe = KIE(ey,gammaE)
    KIe = ey*(ey')*gammaE;
end

== matlab function SAC_RW/Control/ADAPTIVE CONTROLLER/Subsystem1/KPE ==
  data: ey input; Kpe output; gammaE input
function Kpe = KPE(ey,gammaE)
    Kpe = ey*(ey')*gammaE;
end

== matlab function SAC_RW/Control/ADAPTIVE CONTROLLER/Subsystem2/KIX ==
  data: ey input; KIx output; xm input; gammaX input
function KIx = KIX(ey, xm,gammaX)
    KIx = (ey)*(xm')*gammaX;
end

== matlab function SAC_RW/Control/ADAPTIVE CONTROLLER/Subsystem2/KPE ==
  data: ey input; Kpx output; xm input; gammaX input
function Kpx = KPX(ey, xm,gammaX)
    Kpx = (ey)*(xm')*gammaX;
end

== matlab function SAC_RW/Control/ADAPTIVE CONTROLLER/Subsystem3/KIu ==
  data: ey input; um input; KIu output; gammaU input
function KIu = KIU(ey,um,gammaU)
    KIu = ey*(um')*gammaU;
end

== matlab function SAC_RW/Control/ADAPTIVE CONTROLLER/Subsystem3/KPE ==
  data: ey input; KPu output; um input; gammaU input
function KPu = KPU(ey,um,gammaU)
    KPu = ey*(um')*gammaU;
end

== matlab function SAC_RW/Control/ADAPTIVE CONTROLLER/MATLAB Function ==
  data: Tr input; u input; tau output
function tau = torqueGen(Tr, u )

tau = Tr'*u;

end

== matlab function SAC_RW/Control/ADAPTIVE CONTROLLER/Subsystem1/MATLAB Function ==
  data: ey input; KE input; KeEy output
function KeEy = fcn(ey,KE)

KeEy = KE*ey

end
